simulink model "main_model_tube_mpc"  (R2021b)
settings: Solver=ode4  StartTime=0.0  StopTime=3.5  FixedStep=rmpcProps.time_step  RelTol=1e-3
undefined symbols (not defined in the file): driverProps, refTraj, rmpcProps, vehProps
(part 2 of 2)

== system main_model_tube_mpc/Vehicle + Driver Plant Model Nominal/Bicycle Model with Front Steering/Derivatives Of Stability/Subsystem ==
  C1 : Inport
  C2 : Inport  Port=2
  Add : Sum
  Gain : Gain  Gain=-1
  Y_beta : Outport
  wires:
  Add/1 -> Gain/1
  C1/1 -> Add/1
  Gain/1 -> Y_beta/1
  C2/1 -> Add/2

== system main_model_tube_mpc/Vehicle + Driver Plant Model Nominal/Bicycle Model with Front Steering/Derivatives Of Stability/Subsystem1 ==
  a : Inport
  C1 : Inport  Port=2
  b : Inport  Port=3
  C2 : Inport  Port=4
  V : Inport  Port=5
  Add1 : Sum  Inputs=+-
  Divide : Product  Inputs=*/
  Gain1 : Gain  Gain=-1
  Product : Product
  Product1 : Product
  Y_r : Outport
  wires:
  Gain1/1 -> Divide/2
  Product/1 -> Add1/1
  Add1/1 -> Divide/1
  C1/1 -> Product/2
  Product1/1 -> Add1/2
  Divide/1 -> Y_r/1
  b/1 -> Product1/1
  C2/1 -> Product1/2
  V/1 -> Gain1/1
  a/1 -> Product/1

== system main_model_tube_mpc/Vehicle + Driver Plant Model Nominal/Bicycle Model with Front Steering/Derivatives Of Stability/Subsystem2 ==
  a : Inport
  C1 : Inport  Port=2
  b : Inport  Port=3
  C2 : Inport  Port=4
  CMz1 : Inport  Port=5
  CMz2 : Inport  Port=6
  Add2 : Sum  Inputs=++++
  Gain2 : Gain  Gain=-1
  Product2 : Product
  Product3 : Product
  N_beta : Outport
  wires:
  C1/1 -> Product2/2
  Add2/1 -> N_beta/1
  Product3/1 -> Add2/2
  CMz1/1 -> Add2/3
  a/1 -> Gain2/1
  Product2/1 -> Add2/1
  CMz2/1 -> Add2/4
  Gain2/1 -> Product2/1
  b/1 -> Product3/1
  C2/1 -> Product3/2

== system main_model_tube_mpc/Vehicle + Driver Plant Model Nominal/Bicycle Model with Front Steering/Derivatives Of Stability/Subsystem3 ==
  a : Inport
  C1 : Inport  Port=2
  b : Inport  Port=3
  C2 : Inport  Port=4
  CMz1 : Inport  Port=5
  CMz2 : Inport  Port=6
  V : Inport  Port=7
  Add3 : Sum  Inputs=++++
  Divide : Product  Inputs=*/
  Gain3 : Gain  Gain=-1
  Gain4 : Gain  Gain=-1
  Gain5 : Gain  Gain=-1
  Product{4..7} (4 alike) : Product
  Square : Math  Operator=square  SaturateOnIntegerOverflow=on
  Square1 : Math  Operator=square  SaturateOnIntegerOverflow=on
  N_r : Outport
  wires:
  a/1 -> [a], Square/1
  Gain5/1 -> Product7/1
  Gain3/1 -> Product4/1
  Gain4/1 -> Product5/1
  Square1/1 -> Gain4/1
  Product5/1 -> Add3/2
  Product6/1 -> Add3/3
  [b] -> Gain5/1
  Product4/1 -> Add3/1
  Square/1 -> Gain3/1
  Product7/1 -> Add3/4
  CMz1/1 -> Product6/2
  CMz2/1 -> Product7/2
  Add3/1 -> Divide/1
  C1/1 -> Product4/2
  b/1 -> [b], Square1/1
  C2/1 -> Product5/2
  [a] -> Product6/1
  V/1 -> Divide/2
  Divide/1 -> N_r/1

== system main_model_tube_mpc/Vehicle + Driver Plant Model Nominal/Bicycle Model with Front Steering/Derivatives Of Stability/Subsystem4 ==
  a : Inport
  C1 : Inport  Port=2
  CMz1 : Inport  Port=3
  Add : Sum  Inputs=+-
  Product : Product
  N_delta : Outport
  wires:
  a/1 -> Product/1
  Product/1 -> Add/1
  CMz1/1 -> Add/2
  C1/1 -> Product/2
  Add/1 -> N_delta/1

== system main_model_tube_mpc/Vehicle + Driver Plant Model Nominal/Vehicle Trajectory & Footprint/Rotations/x_fl_rotation ==
  x_fl_tr : Inport
  y_fl_tr : Inport  Port=2
  psi : Inport  Port=3
  Add : Sum  Inputs=+-
  Cos : Trigonometry  Operator=cos
  Cos1 : Trigonometry
  Product : Product
  Product1 : Product
  x_fl : Outport
  wires:
  Cos1/1 -> [sin_psi]
  [sin_psi] -> Product1/1
  [cos_psi] -> Product/1
  Product/1 -> Add/1
  Cos/1 -> [cos_psi]
  Product1/1 -> Add/2
  psi/1 -> Cos1/1, Cos/1
  x_fl_tr/1 -> Product/2
  y_fl_tr/1 -> Product1/2
  Add/1 -> x_fl/1

== system main_model_tube_mpc/Vehicle + Driver Plant Model Nominal/Vehicle Trajectory & Footprint/Rotations/x_fr_rotation ==
  x_fr_tr : Inport
  y_fr_tr : Inport  Port=2
  psi : Inport  Port=3
  Add : Sum  Inputs=+-
  Cos : Trigonometry  Operator=cos
  Cos1 : Trigonometry
  Product : Product
  Product1 : Product
  x_fr : Outport
  wires:
  Cos1/1 -> [sin_psi]
  [sin_psi] -> Product1/1
  [cos_psi] -> Product/1
  Product/1 -> Add/1
  Cos/1 -> [cos_psi]
  Product1/1 -> Add/2
  psi/1 -> Cos1/1, Cos/1
  x_fr_tr/1 -> Product/2
  y_fr_tr/1 -> Product1/2
  Add/1 -> x_fr/1

== system main_model_tube_mpc/Vehicle + Driver Plant Model Nominal/Vehicle Trajectory & Footprint/Rotations/x_rl_rotation ==
  x_rl_tr : Inport
  y_rl_tr : Inport  Port=2
  psi : Inport  Port=3
  Add : Sum  Inputs=+-
  Cos : Trigonometry  Operator=cos
  Cos1 : Trigonometry
  Product : Product
  Product1 : Product
  x_rl : Outport
  wires:
  Cos1/1 -> [sin_psi]
  [sin_psi] -> Product1/1
  [cos_psi] -> Product/1
  Product/1 -> Add/1
  Cos/1 -> [cos_psi]
  Product1/1 -> Add/2
  psi/1 -> Cos1/1, Cos/1
  x_rl_tr/1 -> Product/2
  y_rl_tr/1 -> Product1/2
  Add/1 -> x_rl/1

== system main_model_tube_mpc/Vehicle + Driver Plant Model Nominal/Vehicle Trajectory & Footprint/Rotations/x_rr_rotation ==
  x_rr_tr : Inport
  y_rr_tr : Inport  Port=2
  psi : Inport  Port=3
  Add : Sum  Inputs=+-
  Cos : Trigonometry  Operator=cos
  Cos1 : Trigonometry
  Product : Product
  Product1 : Product
  x_rr : Outport
  wires:
  Cos1/1 -> [sin_psi]
  [sin_psi] -> Product1/1
  [cos_psi] -> Product/1
  Product/1 -> Add/1
  Cos/1 -> [cos_psi]
  Product1/1 -> Add/2
  psi/1 -> Cos1/1, Cos/1
  x_rr_tr/1 -> Product/2
  y_rr_tr/1 -> Product1/2
  Add/1 -> x_rr/1

== system main_model_tube_mpc/Vehicle + Driver Plant Model Nominal/Vehicle Trajectory & Footprint/Rotations/y_fl_rotation ==
  x_fl_tr : Inport
  y_fl_tr : Inport  Port=2
  psi : Inport  Port=3
  Add : Sum
  Cos : Trigonometry  Operator=cos
  Cos1 : Trigonometry
  Product : Product
  Product1 : Product
  y_fl : Outport
  wires:
  Cos1/1 -> [sin_psi]
  Product/1 -> Add/1
  Cos/1 -> [cos_psi]
  Product1/1 -> Add/2
  psi/1 -> Cos1/1, Cos/1
  x_fl_tr/1 -> Product/2
  y_fl_tr/1 -> Product1/2
  Add/1 -> y_fl/1
  [cos_psi] -> Product1/1
  [sin_psi] -> Product/1

== system main_model_tube_mpc/Vehicle + Driver Plant Model Nominal/Vehicle Trajectory & Footprint/Rotations/y_fr_rotation ==
  x_fr_tr : Inport
  y_fr_tr : Inport  Port=2
  psi : Inport  Port=3
  Add : Sum
  Cos : Trigonometry  Operator=cos
  Cos1 : Trigonometry
  Product : Product
  Product1 : Product
  y_fr : Outport
  wires:
  Cos1/1 -> [sin_psi]
  Product/1 -> Add/1
  Cos/1 -> [cos_psi]
  Product1/1 -> Add/2
  psi/1 -> Cos1/1, Cos/1
  x_fr_tr/1 -> Product/2
  y_fr_tr/1 -> Product1/2
  Add/1 -> y_fr/1
  [sin_psi] -> Product/1
  [cos_psi] -> Product1/1

== system main_model_tube_mpc/Vehicle + Driver Plant Model Nominal/Vehicle Trajectory & Footprint/Rotations/y_rl_rotation ==
  x_rl_tr : Inport
  y_rl_tr : Inport  Port=2
  psi : Inport  Port=3
  Add : Sum
  Cos : Trigonometry  Operator=cos
  Cos1 : Trigonometry
  Product : Product
  Product1 : Product
  y_rl : Outport
  wires:
  Cos1/1 -> [sin_psi]
  Product/1 -> Add/1
  Cos/1 -> [cos_psi]
  Product1/1 -> Add/2
  psi/1 -> Cos1/1, Cos/1
  x_rl_tr/1 -> Product/2
  y_rl_tr/1 -> Product1/2
  Add/1 -> y_rl/1
  [cos_psi] -> Product1/1
  [sin_psi] -> Product/1

== system main_model_tube_mpc/Vehicle + Driver Plant Model Nominal/Vehicle Trajectory & Footprint/Rotations/y_rr_rotation ==
  x_rr_tr : Inport
  y_rr_tr : Inport  Port=2
  psi : Inport  Port=3
  Add : Sum
  Cos : Trigonometry  Operator=cos
  Cos1 : Trigonometry
  Product : Product
  Product1 : Product
  y_rr : Outport
  wires:
  Cos1/1 -> [sin_psi]
  Product/1 -> Add/1
  Cos/1 -> [cos_psi]
  Product1/1 -> Add/2
  psi/1 -> Cos1/1, Cos/1
  x_rr_tr/1 -> Product/2
  y_rr_tr/1 -> Product1/2
  Add/1 -> y_rr/1
  [cos_psi] -> Product1/1
  [sin_psi] -> Product/1

== matlab function main_model_tube_mpc/Nominal MPC/Controller ==
  data: x0 input; u_ctrl output; U0 input; sv output; rmpcProps parameter; vehProps parameter; driverProps parameter; refTraj parameter
function [u_ctrl,sv] = fcn(x0, U0,rmpcProps,vehProps,driverProps,refTraj)
    u_ctrl=0;
    sv=0;
    coder.extrinsic('steerAssistController_tube');
    [u_ctrl,sv]=steerAssistController_tube(x0,U0,rmpcProps,vehProps,driverProps,refTraj);
end
